simulink model "DstPortLineFilterTest"  (Simulink 6.3)
settings: Solver=ode45  StartTime=0.0  StopTime=10.0  RelTol=1e-3
settings Model: LastModifiedBy=deissenb

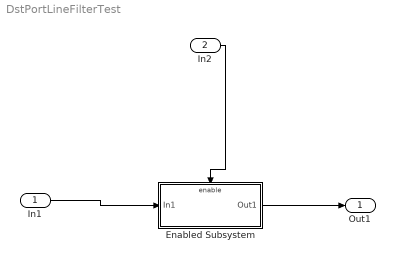
== system DstPortLineFilterTest ==
  In1 : Inport
  In2 : Inport  Port=2
  Enabled Subsystem : Subsystem  TreatAsAtomicUnit=on
  Out1 : Outport
  wires:
  In2/1 -> Enabled Subsystem/Enable
  In1/1 -> Enabled Subsystem/1(In1)
  Enabled Subsystem/1(Out1) -> Out1/1

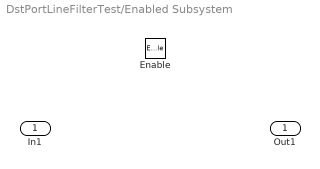
== system DstPortLineFilterTest/Enabled Subsystem ==
  In1 : Inport
  Enable : EnablePort
  Out1 : Outport
